simulink model "TST_AFST_VD"  (R2016b)
settings: Solver=FixedStepDiscrete  StartTime=0.0  StopTime=simTime  FixedStep=sampleTime  RelTol=1e-3
values from neighbouring files (symbols this model uses):
  testCase = 1    [initTST_AFST_VD_001.m]    (also in initTST_AFST_VD_002.m = 2)
libraries: UnitTest_Lib x4, simulink x3
settings Model: Creator=liangyunbo  LastModifiedBy=liangyunbo
settings DebuggingCC: SignalRangeChecking=error

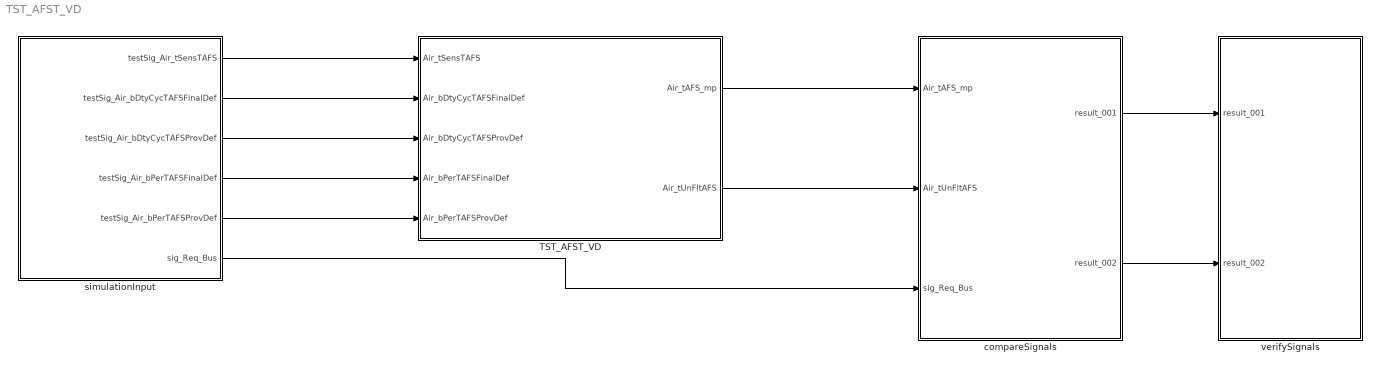
== system TST_AFST_VD ==
  TST_AFST_VD : Subsystem
  compareSignals : Subsystem
  simulationInput : Subsystem
  verifySignals : Subsystem
  wires:
  simulationInput/1(testSig_Air_tSensTAFS) -> TST_AFST_VD/1(Air_tSensTAFS)
  simulationInput/2(testSig_Air_bDtyCycTAFSFinalDef) -> TST_AFST_VD/2(Air_bDtyCycTAFSFinalDef)
  simulationInput/3(testSig_Air_bDtyCycTAFSProvDef) -> TST_AFST_VD/3(Air_bDtyCycTAFSProvDef)
  simulationInput/4(testSig_Air_bPerTAFSFinalDef) -> TST_AFST_VD/4(Air_bPerTAFSFinalDef)
  simulationInput/5(testSig_Air_bPerTAFSProvDef) -> TST_AFST_VD/5(Air_bPerTAFSProvDef)
  TST_AFST_VD/1(Air_tAFS_mp) -> compareSignals/1(Air_tAFS_mp)
  TST_AFST_VD/2(Air_tUnFltAFS) -> compareSignals/2(Air_tUnFltAFS)
  simulationInput/6(sig_Req_Bus) -> compareSignals/3(sig_Req_Bus)
  compareSignals/1(result_001) -> verifySignals/1(result_001)
  compareSignals/2(result_002) -> verifySignals/2(result_002)

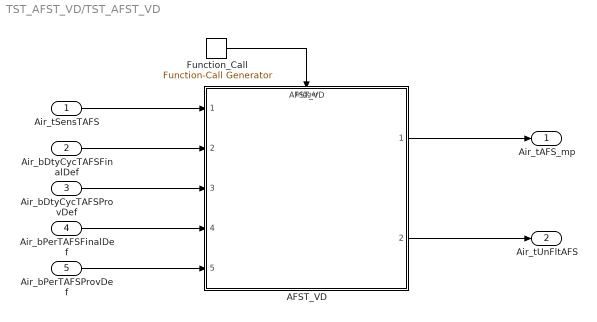
== system TST_AFST_VD/TST_AFST_VD ==
  Air_tSensTAFS : Inport
  Air_bDtyCycTAFSFinalDef : Inport  Port=2
  Air_bDtyCycTAFSProvDef : Inport  Port=3
  Air_bPerTAFSFinalDef : Inport  Port=4
  Air_bPerTAFSProvDef : Inport  Port=5
  AFST_VD : ModelReference  ModelNameDialog=AFST_VD  SimulationMode=Normal  ModelReferenceVersion=1.25  TriggerPortName=function  TriggerPortTriggerType=function-call  TriggerPortStatesWhenEnabling=held
  Function_Call : simulink/Ports & Subsystems/Function-Call Generator  sample_time=sampleTime  numberOfIterations=1
  Air_tAFS_mp : Outport
  Air_tUnFltAFS : Outport  Port=2
  wires:
  Function_Call/1 -> AFST_VD/Trigger
  Air_tSensTAFS/1 -> AFST_VD/1
  Air_bDtyCycTAFSFinalDef/1 -> AFST_VD/2
  Air_bDtyCycTAFSProvDef/1 -> AFST_VD/3
  Air_bPerTAFSFinalDef/1 -> AFST_VD/4
  Air_bPerTAFSProvDef/1 -> AFST_VD/5
  AFST_VD/1 -> Air_tAFS_mp/1
  AFST_VD/2 -> Air_tUnFltAFS/1

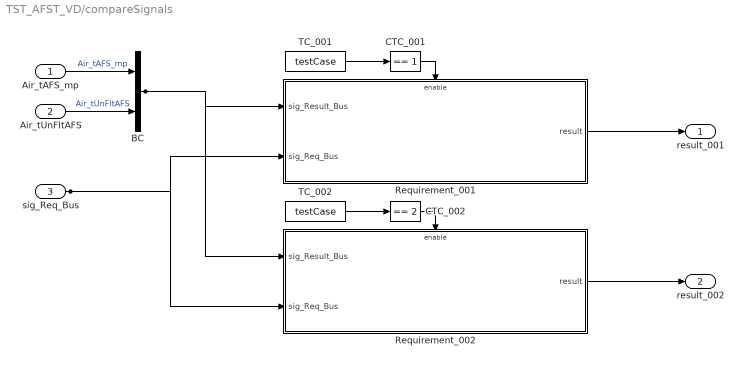
== system TST_AFST_VD/compareSignals ==
  Air_tAFS_mp : Inport
  Air_tUnFltAFS : Inport  Port=2
  sig_Req_Bus : Inport  Port=3
  BC : BusCreator  Inputs=2
  CTC_001 : simulink/Logic and Bit Operations/Compare To Constant  relop===  const=1  OutDataTypeStr=boolean
  CTC_002 : simulink/Logic and Bit Operations/Compare To Constant  relop===  const=2  OutDataTypeStr=boolean
  Requirement_001 : Subsystem
  Requirement_002 : Subsystem
  TC_001 : Constant  Value=testCase
  TC_002 : Constant  Value=testCase
  result_001 : Outport
  result_002 : Outport  Port=2
  wires:
  Air_tAFS_mp/1 -> BC/1  "Air_tAFS_mp"
  Air_tUnFltAFS/1 -> BC/2  "Air_tUnFltAFS"
  TC_001/1 -> CTC_001/1
  CTC_001/1 -> Requirement_001/Enable
  sig_Req_Bus/1 -> Requirement_001/2(sig_Req_Bus), Requirement_002/2(sig_Req_Bus)
  BC/1 -> Requirement_001/1(sig_Result_Bus), Requirement_002/1(sig_Result_Bus)
  Requirement_001/1(result) -> result_001/1
  TC_002/1 -> CTC_002/1
  CTC_002/1 -> Requirement_002/Enable
  Requirement_002/1(result) -> result_002/1

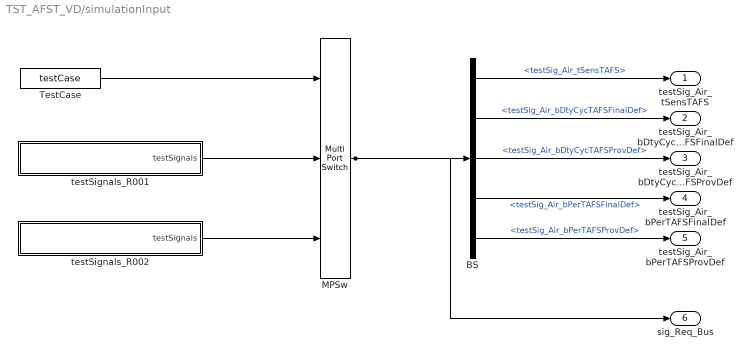
== system TST_AFST_VD/simulationInput ==
  BS : BusSelector  OutputSignals=testSig_Air_tSensTAFS,testSig_Air_bDtyCycTAFSFinalDef,testSig_Air_bDtyCycTAFSProvDef,testSig_Air_bPerTAFSFinalDef,testSig_Air_bPerTAFSProvDef
  MPSw : MultiPortSwitch  Inputs=2  SaturateOnIntegerOverflow=on  InputSameDT=on
  TestCase : Constant  Value=testCase
  testSignals_R001 : Subsystem
  testSignals_R002 : Subsystem
  testSig_Air_tSensTAFS : Outport
  testSig_Air_bDtyCycTAFSFinalDef : Outport  Port=2
  testSig_Air_bDtyCycTAFSProvDef : Outport  Port=3
  testSig_Air_bPerTAFSFinalDef : Outport  Port=4
  testSig_Air_bPerTAFSProvDef : Outport  Port=5
  sig_Req_Bus : Outport  Port=6
  wires:
  BS/1 -> testSig_Air_tSensTAFS/1  "<testSig_Air_tSensTAFS>"
  BS/2 -> testSig_Air_bDtyCycTAFSFinalDef/1  "<testSig_Air_bDtyCycTAFSFinalDef>"
  BS/3 -> testSig_Air_bDtyCycTAFSProvDef/1  "<testSig_Air_bDtyCycTAFSProvDef>"
  BS/4 -> testSig_Air_bPerTAFSFinalDef/1  "<testSig_Air_bPerTAFSFinalDef>"
  BS/5 -> testSig_Air_bPerTAFSProvDef/1  "<testSig_Air_bPerTAFSProvDef>"
  MPSw/1 -> BS/1, sig_Req_Bus/1
  TestCase/1 -> MPSw/1
  testSignals_R001/1(testSignals) -> MPSw/2
  testSignals_R002/1(testSignals) -> MPSw/3

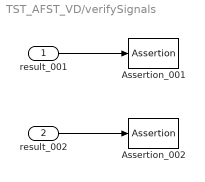
== system TST_AFST_VD/verifySignals ==
  result_001 : Inport
  result_002 : Inport  Port=2
  Assertion_001 : Assertion  Enabled=off
  Assertion_002 : Assertion  Enabled=off
  wires:
  result_001/1 -> Assertion_001/1
  result_002/1 -> Assertion_002/1

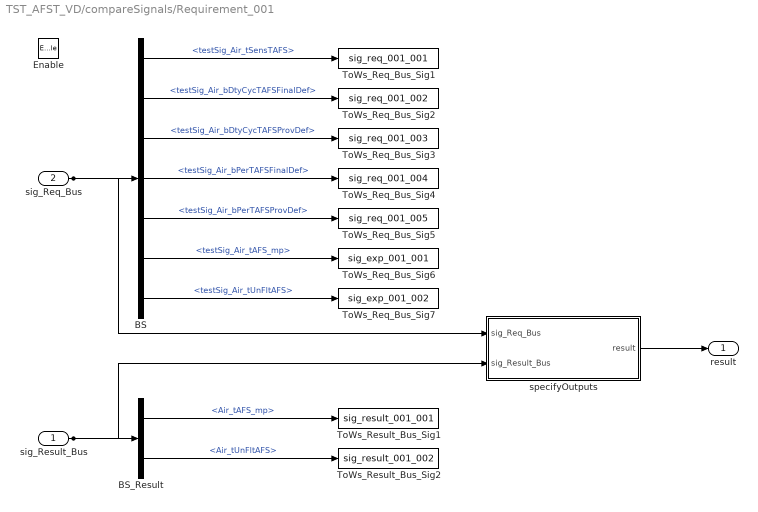
== system TST_AFST_VD/compareSignals/Requirement_001 ==
  sig_Result_Bus : Inport
  sig_Req_Bus : Inport  Port=2
  Enable : EnablePort
  BS : BusSelector  OutputSignals=testSig_Air_tSensTAFS,testSig_Air_bDtyCycTAFSFinalDef,testSig_Air_bDtyCycTAFSProvDef,testSig_Air_bPerTAFSFinalDef,testSig_Air_bPerTAFSProvDef,testSig_Air_tAFS_mp,testSig_Air_tUnFltAFS
  BS_Result : BusSelector  OutputSignals=Air_tAFS_mp,Air_tUnFltAFS
  ToWs_Req_Bus_Sig1 : ToWorkspace  VariableName=sig_req_001_001  SaveFormat=Structure With Time
  ToWs_Req_Bus_Sig2 : ToWorkspace  VariableName=sig_req_001_002  SaveFormat=Structure With Time
  ToWs_Req_Bus_Sig3 : ToWorkspace  VariableName=sig_req_001_003  SaveFormat=Structure With Time
  ToWs_Req_Bus_Sig4 : ToWorkspace  VariableName=sig_req_001_004  SaveFormat=Structure With Time
  ToWs_Req_Bus_Sig5 : ToWorkspace  VariableName=sig_req_001_005  SaveFormat=Structure With Time
  ToWs_Req_Bus_Sig6 : ToWorkspace  VariableName=sig_exp_001_001  SaveFormat=Structure With Time
  ToWs_Req_Bus_Sig7 : ToWorkspace  VariableName=sig_exp_001_002  SaveFormat=Structure With Time
  ToWs_Result_Bus_Sig1 : ToWorkspace  VariableName=sig_result_001_001  SaveFormat=Structure With Time
  ToWs_Result_Bus_Sig2 : ToWorkspace  VariableName=sig_result_001_002  SaveFormat=Structure With Time
  specifyOutputs : Subsystem
  result : Outport
  wires:
  sig_Req_Bus/1 -> BS/1, specifyOutputs/1(sig_Req_Bus)
  BS/1 -> ToWs_Req_Bus_Sig1/1  "<testSig_Air_tSensTAFS>"
  BS/2 -> ToWs_Req_Bus_Sig2/1  "<testSig_Air_bDtyCycTAFSFinalDef>"
  BS/3 -> ToWs_Req_Bus_Sig3/1  "<testSig_Air_bDtyCycTAFSProvDef>"
  BS/4 -> ToWs_Req_Bus_Sig4/1  "<testSig_Air_bPerTAFSFinalDef>"
  BS/5 -> ToWs_Req_Bus_Sig5/1  "<testSig_Air_bPerTAFSProvDef>"
  BS/6 -> ToWs_Req_Bus_Sig6/1  "<testSig_Air_tAFS_mp>"
  BS/7 -> ToWs_Req_Bus_Sig7/1  "<testSig_Air_tUnFltAFS>"
  sig_Result_Bus/1 -> BS_Result/1, specifyOutputs/2(sig_Result_Bus)
  BS_Result/1 -> ToWs_Result_Bus_Sig1/1  "<Air_tAFS_mp>"
  BS_Result/2 -> ToWs_Result_Bus_Sig2/1  "<Air_tUnFltAFS>"
  specifyOutputs/1(result) -> result/1

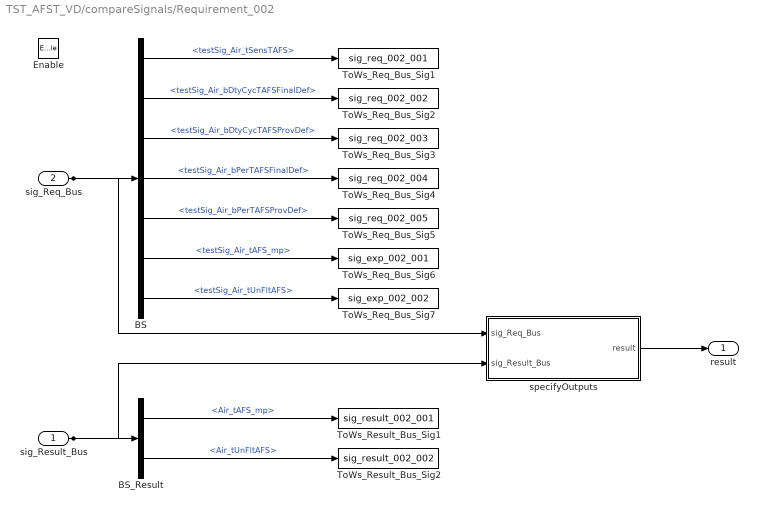
== system TST_AFST_VD/compareSignals/Requirement_002 ==
  sig_Result_Bus : Inport
  sig_Req_Bus : Inport  Port=2
  Enable : EnablePort
  BS : BusSelector  OutputSignals=testSig_Air_tSensTAFS,testSig_Air_bDtyCycTAFSFinalDef,testSig_Air_bDtyCycTAFSProvDef,testSig_Air_bPerTAFSFinalDef,testSig_Air_bPerTAFSProvDef,testSig_Air_tAFS_mp,testSig_Air_tUnFltAFS
  BS_Result : BusSelector  OutputSignals=Air_tAFS_mp,Air_tUnFltAFS
  ToWs_Req_Bus_Sig1 : ToWorkspace  VariableName=sig_req_002_001  SaveFormat=Structure With Time
  ToWs_Req_Bus_Sig2 : ToWorkspace  VariableName=sig_req_002_002  SaveFormat=Structure With Time
  ToWs_Req_Bus_Sig3 : ToWorkspace  VariableName=sig_req_002_003  SaveFormat=Structure With Time
  ToWs_Req_Bus_Sig4 : ToWorkspace  VariableName=sig_req_002_004  SaveFormat=Structure With Time
  ToWs_Req_Bus_Sig5 : ToWorkspace  VariableName=sig_req_002_005  SaveFormat=Structure With Time
  ToWs_Req_Bus_Sig6 : ToWorkspace  VariableName=sig_exp_002_001  SaveFormat=Structure With Time
  ToWs_Req_Bus_Sig7 : ToWorkspace  VariableName=sig_exp_002_002  SaveFormat=Structure With Time
  ToWs_Result_Bus_Sig1 : ToWorkspace  VariableName=sig_result_002_001  SaveFormat=Structure With Time
  ToWs_Result_Bus_Sig2 : ToWorkspace  VariableName=sig_result_002_002  SaveFormat=Structure With Time
  specifyOutputs : Subsystem
  result : Outport
  wires:
  sig_Req_Bus/1 -> BS/1, specifyOutputs/1(sig_Req_Bus)
  BS/1 -> ToWs_Req_Bus_Sig1/1  "<testSig_Air_tSensTAFS>"
  BS/2 -> ToWs_Req_Bus_Sig2/1  "<testSig_Air_bDtyCycTAFSFinalDef>"
  BS/3 -> ToWs_Req_Bus_Sig3/1  "<testSig_Air_bDtyCycTAFSProvDef>"
  BS/4 -> ToWs_Req_Bus_Sig4/1  "<testSig_Air_bPerTAFSFinalDef>"
  BS/5 -> ToWs_Req_Bus_Sig5/1  "<testSig_Air_bPerTAFSProvDef>"
  BS/6 -> ToWs_Req_Bus_Sig6/1  "<testSig_Air_tAFS_mp>"
  BS/7 -> ToWs_Req_Bus_Sig7/1  "<testSig_Air_tUnFltAFS>"
  sig_Result_Bus/1 -> BS_Result/1, specifyOutputs/2(sig_Result_Bus)
  BS_Result/1 -> ToWs_Result_Bus_Sig1/1  "<Air_tAFS_mp>"
  BS_Result/2 -> ToWs_Result_Bus_Sig2/1  "<Air_tUnFltAFS>"
  specifyOutputs/1(result) -> result/1

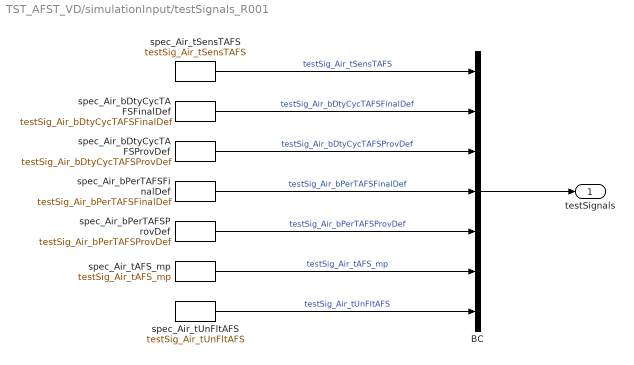
== system TST_AFST_VD/simulationInput/testSignals_R001 ==
  BC : BusCreator  Inputs=7
  spec_Air_bDtyCycTAFSFinalDef : FromWorkspace  VariableName=testSig_Air_bDtyCycTAFSFinalDef  Interpolate=off  OutputAfterFinalValue=Holding final value
  spec_Air_bDtyCycTAFSProvDef : FromWorkspace  VariableName=testSig_Air_bDtyCycTAFSProvDef  Interpolate=off  OutputAfterFinalValue=Holding final value
  spec_Air_bPerTAFSFinalDef : FromWorkspace  VariableName=testSig_Air_bPerTAFSFinalDef  Interpolate=off  OutputAfterFinalValue=Holding final value
  spec_Air_bPerTAFSProvDef : FromWorkspace  VariableName=testSig_Air_bPerTAFSProvDef  Interpolate=off  OutputAfterFinalValue=Holding final value
  spec_Air_tAFS_mp : FromWorkspace  VariableName=testSig_Air_tAFS_mp  Interpolate=off  OutputAfterFinalValue=Holding final value
  spec_Air_tSensTAFS : FromWorkspace  VariableName=testSig_Air_tSensTAFS  Interpolate=off  OutputAfterFinalValue=Holding final value
  spec_Air_tUnFltAFS : FromWorkspace  VariableName=testSig_Air_tUnFltAFS  Interpolate=off  OutputAfterFinalValue=Holding final value
  testSignals : Outport
  wires:
  BC/1 -> testSignals/1
  spec_Air_tSensTAFS/1 -> BC/1  "testSig_Air_tSensTAFS"
  spec_Air_bDtyCycTAFSFinalDef/1 -> BC/2  "testSig_Air_bDtyCycTAFSFinalDef"
  spec_Air_bDtyCycTAFSProvDef/1 -> BC/3  "testSig_Air_bDtyCycTAFSProvDef"
  spec_Air_bPerTAFSFinalDef/1 -> BC/4  "testSig_Air_bPerTAFSFinalDef"
  spec_Air_bPerTAFSProvDef/1 -> BC/5  "testSig_Air_bPerTAFSProvDef"
  spec_Air_tAFS_mp/1 -> BC/6  "testSig_Air_tAFS_mp"
  spec_Air_tUnFltAFS/1 -> BC/7  "testSig_Air_tUnFltAFS"

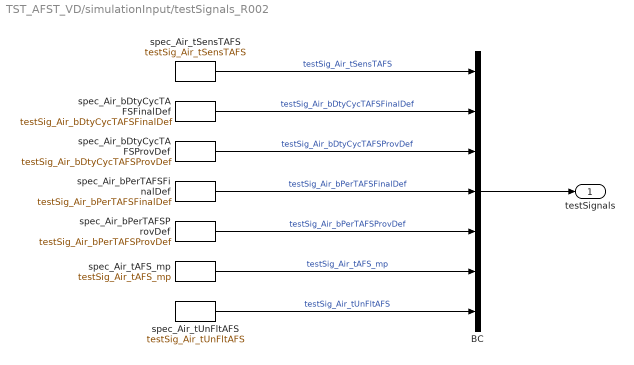
== system TST_AFST_VD/simulationInput/testSignals_R002 ==
  BC : BusCreator  Inputs=7
  spec_Air_bDtyCycTAFSFinalDef : FromWorkspace  VariableName=testSig_Air_bDtyCycTAFSFinalDef  Interpolate=off  OutputAfterFinalValue=Holding final value
  spec_Air_bDtyCycTAFSProvDef : FromWorkspace  VariableName=testSig_Air_bDtyCycTAFSProvDef  Interpolate=off  OutputAfterFinalValue=Holding final value
  spec_Air_bPerTAFSFinalDef : FromWorkspace  VariableName=testSig_Air_bPerTAFSFinalDef  Interpolate=off  OutputAfterFinalValue=Holding final value
  spec_Air_bPerTAFSProvDef : FromWorkspace  VariableName=testSig_Air_bPerTAFSProvDef  Interpolate=off  OutputAfterFinalValue=Holding final value
  spec_Air_tAFS_mp : FromWorkspace  VariableName=testSig_Air_tAFS_mp  Interpolate=off  OutputAfterFinalValue=Holding final value
  spec_Air_tSensTAFS : FromWorkspace  VariableName=testSig_Air_tSensTAFS  Interpolate=off  OutputAfterFinalValue=Holding final value
  spec_Air_tUnFltAFS : FromWorkspace  VariableName=testSig_Air_tUnFltAFS  Interpolate=off  OutputAfterFinalValue=Holding final value
  testSignals : Outport
  wires:
  BC/1 -> testSignals/1
  spec_Air_tSensTAFS/1 -> BC/1  "testSig_Air_tSensTAFS"
  spec_Air_bDtyCycTAFSFinalDef/1 -> BC/2  "testSig_Air_bDtyCycTAFSFinalDef"
  spec_Air_bDtyCycTAFSProvDef/1 -> BC/3  "testSig_Air_bDtyCycTAFSProvDef"
  spec_Air_bPerTAFSFinalDef/1 -> BC/4  "testSig_Air_bPerTAFSFinalDef"
  spec_Air_bPerTAFSProvDef/1 -> BC/5  "testSig_Air_bPerTAFSProvDef"
  spec_Air_tAFS_mp/1 -> BC/6  "testSig_Air_tAFS_mp"
  spec_Air_tUnFltAFS/1 -> BC/7  "testSig_Air_tUnFltAFS"

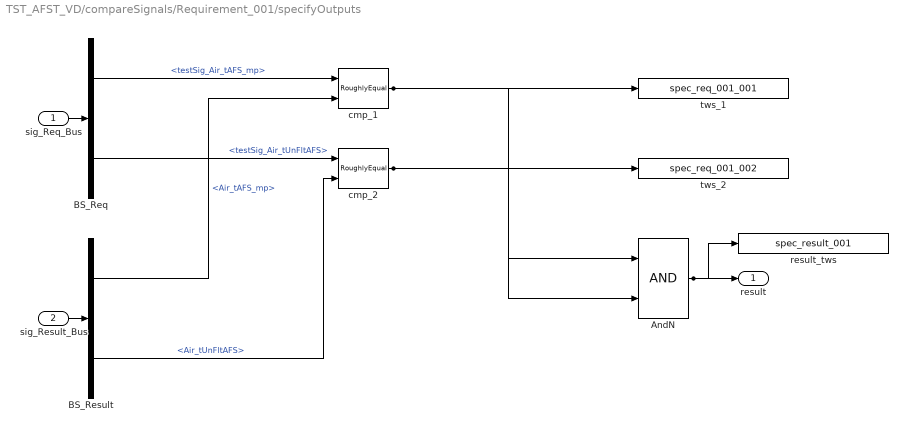
== system TST_AFST_VD/compareSignals/Requirement_001/specifyOutputs ==
  sig_Req_Bus : Inport
  sig_Result_Bus : Inport  Port=2
  AndN : Logic
  BS_Req : BusSelector  OutputSignals=testSig_Air_tAFS_mp,testSig_Air_tUnFltAFS
  BS_Result : BusSelector  OutputSignals=Air_tAFS_mp,Air_tUnFltAFS
  cmp_1 : UnitTest_Lib/RoughlyEqual  slope=0.1
  cmp_2 : UnitTest_Lib/RoughlyEqual  slope=0.1
  result_tws : ToWorkspace  VariableName=spec_result_001
  tws_1 : ToWorkspace  VariableName=spec_req_001_001
  tws_2 : ToWorkspace  VariableName=spec_req_001_002
  result : Outport
  wires:
  sig_Req_Bus/1 -> BS_Req/1
  sig_Result_Bus/1 -> BS_Result/1
  AndN/1 -> result/1, result_tws/1
  BS_Req/1 -> cmp_1/1  "<testSig_Air_tAFS_mp>"
  BS_Result/1 -> cmp_1/2  "<Air_tAFS_mp>"
  cmp_1/1 -> tws_1/1, AndN/1
  BS_Req/2 -> cmp_2/1  "<testSig_Air_tUnFltAFS>"
  BS_Result/2 -> cmp_2/2  "<Air_tUnFltAFS>"
  cmp_2/1 -> tws_2/1, AndN/2

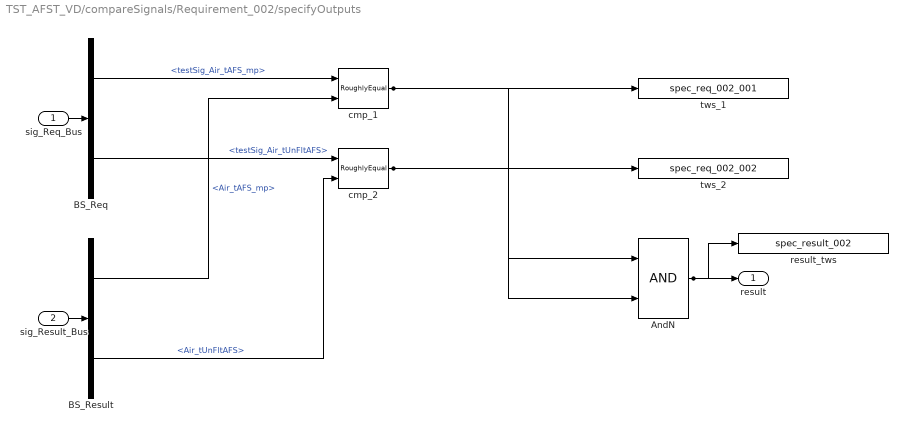
== system TST_AFST_VD/compareSignals/Requirement_002/specifyOutputs ==
  sig_Req_Bus : Inport
  sig_Result_Bus : Inport  Port=2
  AndN : Logic
  BS_Req : BusSelector  OutputSignals=testSig_Air_tAFS_mp,testSig_Air_tUnFltAFS
  BS_Result : BusSelector  OutputSignals=Air_tAFS_mp,Air_tUnFltAFS
  cmp_1 : UnitTest_Lib/RoughlyEqual  slope=0.1
  cmp_2 : UnitTest_Lib/RoughlyEqual  slope=0.1
  result_tws : ToWorkspace  VariableName=spec_result_002
  tws_1 : ToWorkspace  VariableName=spec_req_002_001
  tws_2 : ToWorkspace  VariableName=spec_req_002_002
  result : Outport
  wires:
  sig_Req_Bus/1 -> BS_Req/1
  sig_Result_Bus/1 -> BS_Result/1
  AndN/1 -> result/1, result_tws/1
  BS_Req/1 -> cmp_1/1  "<testSig_Air_tAFS_mp>"
  BS_Result/1 -> cmp_1/2  "<Air_tAFS_mp>"
  cmp_1/1 -> tws_1/1, AndN/1
  BS_Req/2 -> cmp_2/1  "<testSig_Air_tUnFltAFS>"
  BS_Result/2 -> cmp_2/2  "<Air_tUnFltAFS>"
  cmp_2/1 -> tws_2/1, AndN/2
